simulink model "mult_1"  (R2023a)
settings: Solver=FixedStepDiscrete  StartTime=0.0  StopTime=10.0  RelTol=1e-3
undefined symbols (not defined in the file): dt
libraries: simulink x1
settings Model: DataTypeOverride=Off  Creator=szymadej  LastModifiedBy=szymadej
settings OptimizationCC: BlockReduction=off  ConditionallyExecuteInputs=off  DefaultParameterBehavior=Inlined  InheritOutputTypeSmallerThanSingle=on
settings DebuggingCC: AlgebraicLoopMsg=error  SingleTaskRateTransMsg=error  UnconnectedInputMsg=warning  UnconnectedOutputMsg=warning  UnconnectedLineMsg=warning
settings HardwareCC: ProdBitPerPointer=32  ProdBitPerSizeT=32  ProdBitPerPtrDiffT=32  ProdLargestAtomicFloat=None  ProdIntDivRoundTo=Undefined  ProdEndianess=Unspecified  ProdWordSize=32  ProdHWDeviceType=ASIC/FPGA->ASIC/FPGA  TargetBitPerLong=64  TargetBitPerPointer=64  TargetBitPerSizeT=64  TargetBitPerPtrDiffT=64  TargetLongLongMode=on  TargetIntDivRoundTo=Zero  TargetEndianess=LittleEndian  TargetWordSize=64  TargetHWDeviceType=Custom Processor->MATLAB Host Computer  ProdEqTarget=off

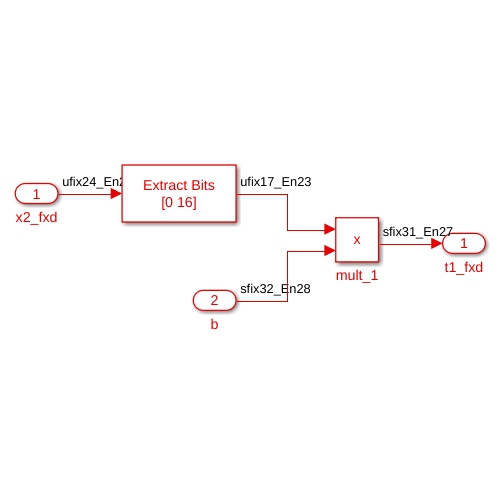
[thumbnail: Simulink's stored preview of the top-level diagram]
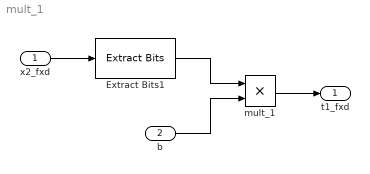
== system mult_1 ==
  x2_fxd : Inport  OutDataTypeStr=fixdt(dt.x_fxd.s,dt.x_fxd.w,dt.x_fxd.f)
  b : Inport  Port=2  OutDataTypeStr=fixdt(dt.coeff_fxd.s,dt.coeff_fxd.w,dt.coeff_fxd.f)
  Extract Bits1 : simulink/Logic and Bit Operations/Extract Bits  bitsToExtract=Range of bits  numBits=17  bitIdxRange=[0 dt.x2_fxd.w-1]  outScalingMode=Preserve fixed-point scaling
  mult_1 : Product  OutDataTypeStr=fixdt(dt.t1_fxd.s,dt.t1_fxd.w,dt.t1_fxd.f)
  t1_fxd : Outport
  wires:
  x2_fxd/1 -> Extract Bits1/1
  mult_1/1 -> t1_fxd/1
  b/1 -> mult_1/2
  Extract Bits1/1 -> mult_1/1
